simulink model "deep_pp"  (R2025b)
settings: Solver=FixedStepAuto  StartTime=0.0  StopTime=300  FixedStep=.01  RelTol=1e-3
undefined symbols (not defined in the file or in its folder): battery_builder_rtmsupport, gcbh
libraries: Batteries_lib x15, nesl_utility x5, fl_lib x4, ee_lib x1
(part 1 of 2)
settings Model: Creator=nhamb  LastModifiedBy=nhamb

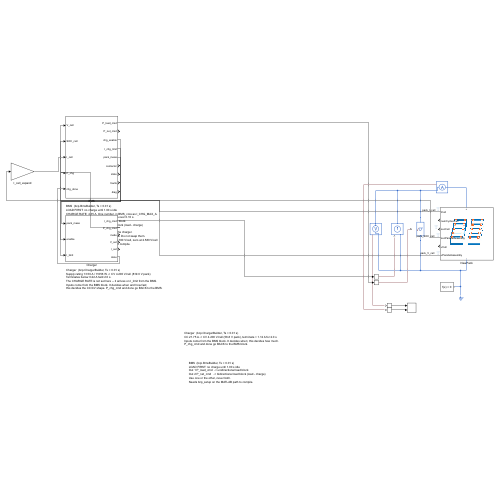
[thumbnail: Simulink's stored preview of the top-level diagram]
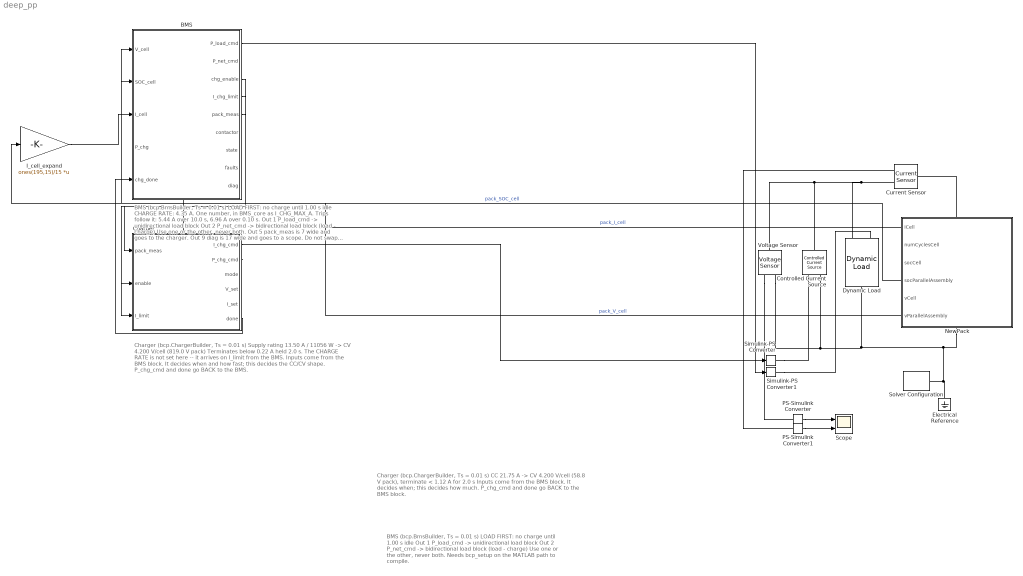
== system deep_pp ==
  note: BMS  (bcp.BmsBuilder, Ts = 0.01 s)
      | LOAD FIRST: no charge until 1.00 s idle
      | Out 1 P_load_cmd  -> unidirectional load block
      | Out 2 P_net_cmd   -> bidirectional load block (load - charge)
      | Use one or the other, never both.
      | Needs bcp_setup on the MATLAB path to compile.
  note: Charger  (bcp.ChargerBuilder, Ts = 0.01 s)
      | CC 21.75 A -> CV 4.200 V/cell (58.8 V pack), terminate < 1.12 A for 2.0 s
      | Inputs come from the BMS block. It decides when; this decides how much.
      | P_chg_cmd and done go BACK to the BMS block.
  note: BMS  (bcp.BmsBuilder, Ts = 0.01 s)
      | LOAD FIRST: no charge until 1.00 s idle
      | CHARGE RATE: 4.35 A. One number, in BMS_core as I_CHG_MAX_A.
      |   Trips follow it: 5.44 A over 10.0 s, 6.96 A over 0.10 s.
      | Out 1 P_load_cmd  -> unidirectional load block
      | Out 2 P_net_cmd   -> bidirectional load block (load - charge)
      | Use one or the other, never both.
      | Out 5 pack_meas is 7 wide and goes to the charger.
      | Out 9 diag is 17 wide and goes to a scope. Do not swap them.
      | DISCHARGE LIMITER: full load above 2.780 V/cell, zero at 2.580 V/cell
      | Needs bcp_setup on the MATLAB path to compile.
  note: Charger  (bcp.ChargerBuilder, Ts = 0.01 s)
      | Supply rating 13.50 A / 11056 W -> CV 4.200 V/cell (819.0 V pack)
      | Terminates below 0.22 A held 2.0 s.
      | The CHARGE RATE is not set here -- it arrives on I_limit from the BMS.
      | Inputs come from the BMS block. It decides when and how fast;
      | this decides the CC/CV shape. P_chg_cmd and done go BACK to the BMS.
  BMS : Subsystem
  Charger : Subsystem
  Controlled Current Source : fl_lib/Electrical/Electrical Sources/Controlled Current Source
  Current Sensor : fl_lib/Electrical/Electrical Sensors/Current Sensor
  Dynamic Load : ee_lib/Passive/Dynamic Load  load_type=ee.enum.dc_ac.dc  min_supply_voltage=20 V  pow_min=1e-3 W  G_reverse=1e-6 S  deltaV=1e-3 V  f0=60 Hz  Vrms_min=200 V  tau=0.01 s  Vrms_ini=300 V  Vang_ini=0 deg
      settings: InternalSimscapePortConfiguration="{\"Bottom\":[],\"Left\":[{\"id\":\"p\",\"label\":\"+\",\"type\":\"foundation.electrical.electrical\"}],\"Right\":[{\"id\":\"n\",\"label\":\"-\",\"type\":\"foundation.electrical.electrical\"}],\"Top\":[{\"id\":\"P\",\"label\":\"P\",\"type\":\"input\"}]}"
  Electrical Reference : fl_lib/Electrical/Electrical Elements/Electrical Reference
  I_cell_expand : Gain  Gain=ones(195,15)/15  Multiplication=Matrix(K*u)
  NewPack : Subsystem  LoadFcn=battery_builder_rtmsupport('loadfcn',gcbh);
      settings: CopyFcn=battery_builder_rtmsupport('copyfcn',gcbh);  PreCopyFcn=battery_builder_rtmsupport('precopyfcn',gcbh);  PreDeleteFcn=battery_builder_rtmsupport('predeletefcn',gcbh);  PortSchema="{\"entries\":[{\"content\":{\"sides\":[{\"content\":{\"connectorIds\":[\"LConn1\"]},\"type\":\"ConnectorPlacement.EquallySpacedRectSide\",\"uuid\":\"639f1e3e-b529-4ef3-8a0e-59dadedc297f\"},{\"content\":{\"connectorIds\":[\"RConn1\"],\"side\":\"RIGHT\"},\"type\":\"ConnectorPlacement.EquallySpacedRectSide\",\"uuid\":\"fd02ecdf-1885-4056-8ffe-a1dd80f7e2bb\"},{\"content\":{\"side\":\"TOP\"},\"type\":\"ConnectorPlacement.EquallySpacedRectSide\",\"uuid\":\"7ee78b50-8b8e-447f-8754-7e3c87fbecdf\"},{\"content\":{\"connectorIds\":[\"Out1\",\"Out2\",\"Out3\",\"Out4\",\"Out5\",\"Out6\"],\"side\":\"BOTTOM\"},\"type\":\"ConnectorPlacement.EquallySpacedRectSide\",\"uuid\":\"bf99fb64-3b35-4929-842b-dc936d21827d\"}]},\"type\":\"ConnectorPlacement.EquallySpacedConnector\",\"uuid\":\"bfe7ef6e-8305-4395-9b95-13fe458d8955\"}],\"packageUris\":[\"http://schema.mathworks.com/mf0/Connector/R2020b\"],\"version\":\"1.0\"}"
      mask Display: image('$imagefile')
  PS-Simulink Converter : nesl_utility/PS-Simulink Converter  PhysicalDomain=network_engine_domain  SubClassName=ps_output  LeftPortType=input  RightPortType=output  PseudoPeriodic=off  Frequencies=[]  VectorFormat=inherit  Unit=inherit  AffineConversion=off
  PS-Simulink Converter1 : nesl_utility/PS-Simulink Converter  PhysicalDomain=network_engine_domain  SubClassName=ps_output  LeftPortType=input  RightPortType=output  PseudoPeriodic=off  Frequencies=[]  VectorFormat=inherit  Unit=inherit  AffineConversion=off
  Scope : Scope  NumInputPorts=2
      settings: ActiveDisplayYMinimum=41.312958628712209  ActiveDisplayYMaximum=167.00529821946185
  Simulink-PS Converter : nesl_utility/Simulink-PS Converter  PhysicalDomain=network_engine_domain  SubClassName=ps_input  LeftPortType=input  RightPortType=output  PseudoPeriodic=off  Frequencies=[]  NoiseDistribution=none  NoiseParameters=[]  Unit=1  AffineConversion=off  FilteringAndDerivatives=provide  SimscapeFilterOrder=1  InputFilterTimeConstant=0.001  UdotUserProvided=0
  Simulink-PS Converter1 : nesl_utility/Simulink-PS Converter  PhysicalDomain=network_engine_domain  SubClassName=ps_input  LeftPortType=input  RightPortType=output  PseudoPeriodic=off  Frequencies=[]  NoiseDistribution=none  NoiseParameters=[]  Unit=1  AffineConversion=off  FilteringAndDerivatives=provide  SimscapeFilterOrder=1  InputFilterTimeConstant=0.001  UdotUserProvided=0
  Solver Configuration : nesl_utility/Solver Configuration  PhysicalDomain=network_engine_domain  SubClassName=solver  LeftPortType=input  RightPortType=generic  Tones=[]  Harmonics=[]  SimulateNoise=off  Profile=off  UseLocalSampling=off  EnableSwitchedLinearOptims=on  FrequencyDomain=off  UseCCode=off  RelTol=0.001  AbsTol=0.001  MinStep=1e-09  ToWorkspace=off  RevertToSquareIcSolve=off  NumHomotopyIterations=100  PhasorMode=off  PhasorModeNumHarmonics=1  ConsistencySolver=NEWTON_XTOL_AFTER_FTOL  IndexReductionMethod=DerivativeReplacement  DoDC=off  ResidualTolerance=1e-09  ConsistencyTolSource=GLOBAL  ConsistencyAbsTol=0.001  ConsistencyRelTol=0.001  ConsistencyTolFactor=0.001  UseLocalSolver=off  LocalSolverChoice=NE_BACKWARD_EULER_ADVANCER  ResolveIndetEquations=on  FunctionEvalNumThread=1  LocalSolverSampleTime=0.001  DoFixedCost=off  MaxNonlinIter=3  MaxModeIter=2  ComputeImpulses=off  ImpulseIterations=2  LinearAlgebra=auto  LinearAlgebraNumThread=0  EquationFormulation=NE_TIME_EF  DelaysMemoryBudget=1024  AutomaticFiltering=on  FilteringTimeConstant=0.001  PartitionStorageMethod=AS_NEEDED  PartitionMemoryBudget=1024  PartitionMethod=ROBUST  MultibodyUseLocalSolver=off  MultibodyLocalSolverChoice=ODE1  MultibodyLocalSolverSampleTime=0.001
  Voltage Sensor : fl_lib/Electrical/Electrical Sensors/Voltage Sensor
  wires:
  PS-Simulink Converter1/1 -> Scope/2
  PS-Simulink Converter/1 -> Scope/1
  BMS/5(pack_meas) -> Charger/1(pack_meas)
  BMS/3(chg_enable) -> Charger/2(enable)
  BMS/4(I_chg_limit) -> Charger/3(I_limit)
  Charger/2(P_chg_cmd) -> BMS/4(P_chg)
  Charger/6(done) -> BMS/5(chg_done)
  NewPack/1(iCell) -> I_cell_expand/1  "pack_I_cell"
  I_cell_expand/1 -> BMS/3(I_cell)
  NewPack/6(vParallelAssembly) -> BMS/1(V_cell)  "pack_V_cell"
  NewPack/4(socParallelAssembly) -> BMS/2(SOC_cell)  "pack_SOC_cell"
  BMS/1(P_load_cmd) -> Simulink-PS Converter1/1
  Charger/1(I_chg_cmd) -> Simulink-PS Converter/1
  connections:
  Controlled Current Source/RConn2 -- Solver Configuration/RConn1 -- Electrical Reference/LConn1 -- NewPack/RConn1 -- Dynamic Load/RConn1 -- Voltage Sensor/RConn2
  Current Sensor/RConn2 -- Dynamic Load/LConn1 -- Voltage Sensor/LConn1 -- Controlled Current Source/LConn1
  NewPack/LConn1 -- Current Sensor/LConn1
  Simulink-PS Converter/RConn1 -- Controlled Current Source/RConn1
  Simulink-PS Converter1/RConn1 -- Dynamic Load/LConn2
  Voltage Sensor/RConn1 -- PS-Simulink Converter/LConn1
  Current Sensor/RConn1 -- PS-Simulink Converter1/LConn1

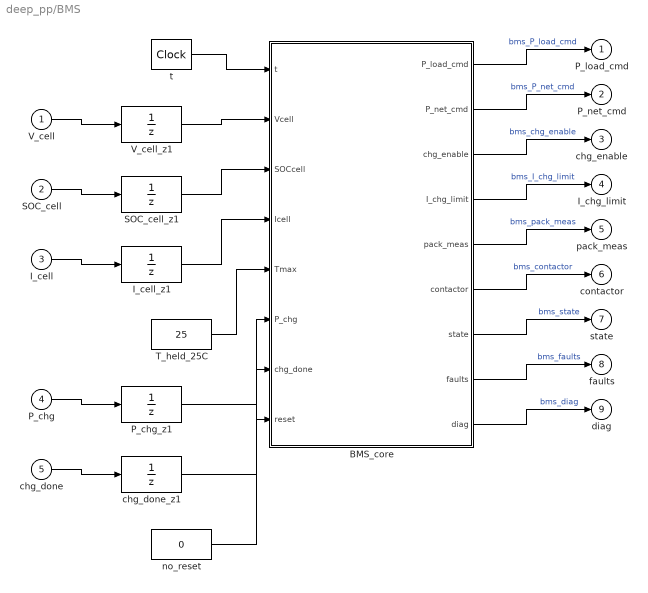
== system deep_pp/BMS ==
  V_cell : Inport
  SOC_cell : Inport  Port=2
  I_cell : Inport  Port=3
  P_chg : Inport  Port=4
  chg_done : Inport  Port=5
  BMS_core : MATLAB Function  TreatAsAtomicUnit=on
  I_cell_z1 : UnitDelay  SampleTime=0.01  HasFrameUpgradeWarning=on
  P_chg_z1 : UnitDelay  SampleTime=0.01  HasFrameUpgradeWarning=on
  SOC_cell_z1 : UnitDelay  InitialCondition=0.5  SampleTime=0.01  HasFrameUpgradeWarning=on
  T_held_25C : Constant  Value=25
  V_cell_z1 : UnitDelay  InitialCondition=3.575  SampleTime=0.01  HasFrameUpgradeWarning=on
  chg_done_z1 : UnitDelay  SampleTime=0.01  HasFrameUpgradeWarning=on
  no_reset : Constant  Value=0
  t : DigitalClock  SampleTime=0.01
  P_load_cmd : Outport
  P_net_cmd : Outport  Port=2
  chg_enable : Outport  Port=3
  I_chg_limit : Outport  Port=4
  pack_meas : Outport  Port=5
  contactor : Outport  Port=6
  state : Outport  Port=7
  faults : Outport  Port=8
  diag : Outport  Port=9
  wires:
  t/1 -> BMS_core/1(t)
  V_cell/1 -> V_cell_z1/1
  V_cell_z1/1 -> BMS_core/2(Vcell)
  SOC_cell/1 -> SOC_cell_z1/1
  SOC_cell_z1/1 -> BMS_core/3(SOCcell)
  I_cell/1 -> I_cell_z1/1
  I_cell_z1/1 -> BMS_core/4(Icell)
  T_held_25C/1 -> BMS_core/5(Tmax)
  P_chg/1 -> P_chg_z1/1
  P_chg_z1/1 -> BMS_core/6(P_chg)
  chg_done/1 -> chg_done_z1/1
  chg_done_z1/1 -> BMS_core/7(chg_done)
  no_reset/1 -> BMS_core/8(reset)
  BMS_core/1(P_load_cmd) -> P_load_cmd/1  "bms_P_load_cmd"
  BMS_core/2(P_net_cmd) -> P_net_cmd/1  "bms_P_net_cmd"
  BMS_core/3(chg_enable) -> chg_enable/1  "bms_chg_enable"
  BMS_core/4(I_chg_limit) -> I_chg_limit/1  "bms_I_chg_limit"
  BMS_core/5(pack_meas) -> pack_meas/1  "bms_pack_meas"
  BMS_core/6(contactor) -> contactor/1  "bms_contactor"
  BMS_core/7(state) -> state/1  "bms_state"
  BMS_core/8(faults) -> faults/1  "bms_faults"
  BMS_core/9(diag) -> diag/1  "bms_diag"

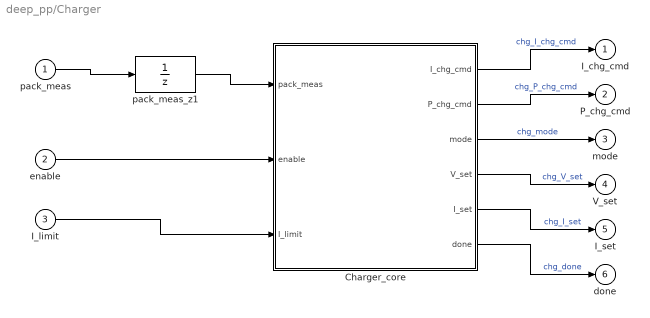
== system deep_pp/Charger ==
  pack_meas : Inport
  enable : Inport  Port=2
  I_limit : Inport  Port=3
  Charger_core : MATLAB Function  TreatAsAtomicUnit=on
  pack_meas_z1 : UnitDelay  InitialCondition=[819;4.2;4.2;1;1;1;0]  SampleTime=0.01  HasFrameUpgradeWarning=on
  I_chg_cmd : Outport
  P_chg_cmd : Outport  Port=2
  mode : Outport  Port=3
  V_set : Outport  Port=4
  I_set : Outport  Port=5
  done : Outport  Port=6
  wires:
  pack_meas/1 -> pack_meas_z1/1
  pack_meas_z1/1 -> Charger_core/1(pack_meas)
  enable/1 -> Charger_core/2(enable)
  I_limit/1 -> Charger_core/3(I_limit)
  Charger_core/1(I_chg_cmd) -> I_chg_cmd/1  "chg_I_chg_cmd"
  Charger_core/2(P_chg_cmd) -> P_chg_cmd/1  "chg_P_chg_cmd"
  Charger_core/3(mode) -> mode/1  "chg_mode"
  Charger_core/4(V_set) -> V_set/1  "chg_V_set"
  Charger_core/5(I_set) -> I_set/1  "chg_I_set"
  Charger_core/6(done) -> done/1  "chg_done"

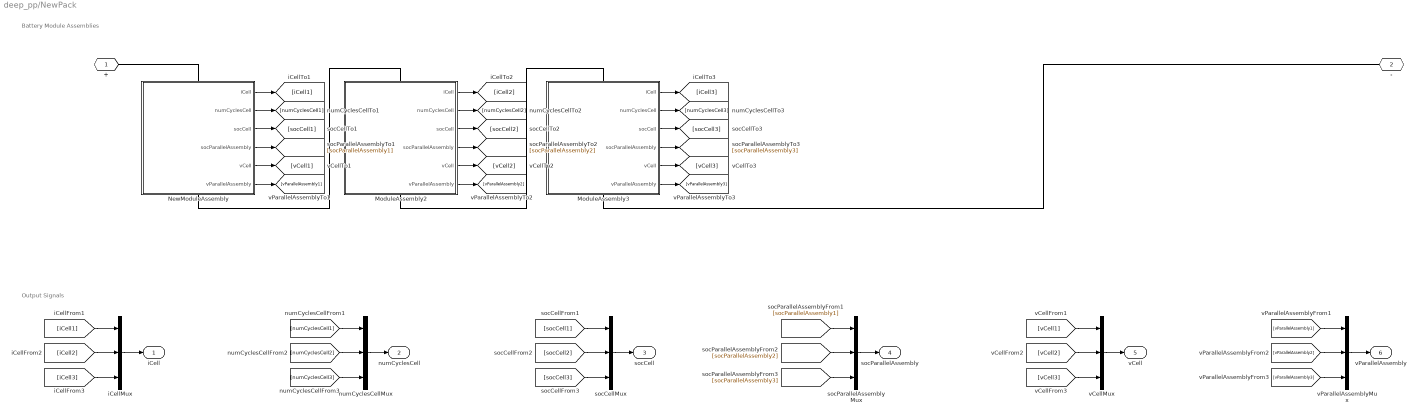
== system deep_pp/NewPack ==
  note: Output Signals
  note: Battery Module Assemblies
  ModuleAssembly2 : Subsystem  LoadFcn=battery_builder_rtmsupport('loadfcn',gcbh);
      settings: CopyFcn=battery_builder_rtmsupport('copyfcn',gcbh);  PreCopyFcn=battery_builder_rtmsupport('precopyfcn',gcbh);  PreDeleteFcn=battery_builder_rtmsupport('predeletefcn',gcbh);  PortSchema="{\"entries\":[{\"content\":{\"sides\":[{\"content\":{\"connectorIds\":[\"LConn1\"]},\"type\":\"ConnectorPlacement.EquallySpacedRectSide\",\"uuid\":\"639f1e3e-b529-4ef3-8a0e-59dadedc297f\"},{\"content\":{\"connectorIds\":[\"RConn1\"],\"side\":\"RIGHT\"},\"type\":\"ConnectorPlacement.EquallySpacedRectSide\",\"uuid\":\"fd02ecdf-1885-4056-8ffe-a1dd80f7e2bb\"},{\"content\":{\"side\":\"TOP\"},\"type\":\"ConnectorPlacement.EquallySpacedRectSide\",\"uuid\":\"7ee78b50-8b8e-447f-8754-7e3c87fbecdf\"},{\"content\":{\"connectorIds\":[\"Out1\",\"Out2\",\"Out3\",\"Out4\",\"Out5\",\"Out6\"],\"side\":\"BOTTOM\"},\"type\":\"ConnectorPlacement.EquallySpacedRectSide\",\"uuid\":\"6ddc3ac7-a805-4d8e-a52b-67f31048dafb\"}]},\"type\":\"ConnectorPlacement.EquallySpacedConnector\",\"uuid\":\"bfe7ef6e-8305-4395-9b95-13fe458d8955\"}],\"packageUris\":[\"http://schema.mathworks.com/mf0/Connector/R2020b\"],\"version\":\"1.0\"}"
      mask Display: image('$imagefile')
  ModuleAssembly3 : Subsystem  LoadFcn=battery_builder_rtmsupport('loadfcn',gcbh);
      settings: CopyFcn=battery_builder_rtmsupport('copyfcn',gcbh);  PreCopyFcn=battery_builder_rtmsupport('precopyfcn',gcbh);  PreDeleteFcn=battery_builder_rtmsupport('predeletefcn',gcbh);  PortSchema="{\"entries\":[{\"content\":{\"sides\":[{\"content\":{\"connectorIds\":[\"LConn1\"]},\"type\":\"ConnectorPlacement.EquallySpacedRectSide\",\"uuid\":\"639f1e3e-b529-4ef3-8a0e-59dadedc297f\"},{\"content\":{\"connectorIds\":[\"RConn1\"],\"side\":\"RIGHT\"},\"type\":\"ConnectorPlacement.EquallySpacedRectSide\",\"uuid\":\"fd02ecdf-1885-4056-8ffe-a1dd80f7e2bb\"},{\"content\":{\"side\":\"TOP\"},\"type\":\"ConnectorPlacement.EquallySpacedRectSide\",\"uuid\":\"7ee78b50-8b8e-447f-8754-7e3c87fbecdf\"},{\"content\":{\"connectorIds\":[\"Out1\",\"Out2\",\"Out3\",\"Out4\",\"Out5\",\"Out6\"],\"side\":\"BOTTOM\"},\"type\":\"ConnectorPlacement.EquallySpacedRectSide\",\"uuid\":\"6ddc3ac7-a805-4d8e-a52b-67f31048dafb\"}]},\"type\":\"ConnectorPlacement.EquallySpacedConnector\",\"uuid\":\"bfe7ef6e-8305-4395-9b95-13fe458d8955\"}],\"packageUris\":[\"http://schema.mathworks.com/mf0/Connector/R2020b\"],\"version\":\"1.0\"}"
      mask Display: image('moduleAssembly_1.JPG');
  NewModuleAssembly : Subsystem  LoadFcn=battery_builder_rtmsupport('loadfcn',gcbh);
      settings: CopyFcn=battery_builder_rtmsupport('copyfcn',gcbh);  PreCopyFcn=battery_builder_rtmsupport('precopyfcn',gcbh);  PreDeleteFcn=battery_builder_rtmsupport('predeletefcn',gcbh);  PortSchema="{\"entries\":[{\"content\":{\"sides\":[{\"content\":{\"connectorIds\":[\"LConn1\"]},\"type\":\"ConnectorPlacement.EquallySpacedRectSide\",\"uuid\":\"639f1e3e-b529-4ef3-8a0e-59dadedc297f\"},{\"content\":{\"connectorIds\":[\"RConn1\"],\"side\":\"RIGHT\"},\"type\":\"ConnectorPlacement.EquallySpacedRectSide\",\"uuid\":\"fd02ecdf-1885-4056-8ffe-a1dd80f7e2bb\"},{\"content\":{\"side\":\"TOP\"},\"type\":\"ConnectorPlacement.EquallySpacedRectSide\",\"uuid\":\"7ee78b50-8b8e-447f-8754-7e3c87fbecdf\"},{\"content\":{\"connectorIds\":[\"Out1\",\"Out2\",\"Out3\",\"Out4\",\"Out5\",\"Out6\"],\"side\":\"BOTTOM\"},\"type\":\"ConnectorPlacement.EquallySpacedRectSide\",\"uuid\":\"6ddc3ac7-a805-4d8e-a52b-67f31048dafb\"}]},\"type\":\"ConnectorPlacement.EquallySpacedConnector\",\"uuid\":\"bfe7ef6e-8305-4395-9b95-13fe458d8955\"}],\"packageUris\":[\"http://schema.mathworks.com/mf0/Connector/R2020b\"],\"version\":\"1.0\"}"
      mask Display: image('moduleAssembly_2.JPG');
  iCellMux : Mux  Inputs=3
  numCyclesCellMux : Mux  Inputs=3
  socCellMux : Mux  Inputs=3
  socParallelAssemblyMux : Mux  Inputs=3
  vCellMux : Mux  Inputs=3
  vParallelAssemblyMux : Mux  Inputs=3
  + : PMIOPort  Side=Left
  - : PMIOPort  Port=2  Side=Right
  iCell : Outport
  numCyclesCell : Outport  Port=2
  socCell : Outport  Port=3
  socParallelAssembly : Outport  Port=4
  vCell : Outport  Port=5
  vParallelAssembly : Outport  Port=6
  wires:
  [vParallelAssembly3] -> vParallelAssemblyMux/3
  ModuleAssembly3/6(vParallelAssembly) -> [vParallelAssembly3]
  [vCell3] -> vCellMux/3
  ModuleAssembly3/5(vCell) -> [vCell3]
  [socParallelAssembly3] -> socParallelAssemblyMux/3
  ModuleAssembly3/4(socParallelAssembly) -> [socParallelAssembly3]
  [socCell3] -> socCellMux/3
  ModuleAssembly3/3(socCell) -> [socCell3]
  [numCyclesCell3] -> numCyclesCellMux/3
  ModuleAssembly3/2(numCyclesCell) -> [numCyclesCell3]
  [iCell3] -> iCellMux/3
  ModuleAssembly3/1(iCell) -> [iCell3]
  [vParallelAssembly2] -> vParallelAssemblyMux/2
  ModuleAssembly2/6(vParallelAssembly) -> [vParallelAssembly2]
  [vCell2] -> vCellMux/2
  ModuleAssembly2/5(vCell) -> [vCell2]
  [socParallelAssembly2] -> socParallelAssemblyMux/2
  ModuleAssembly2/4(socParallelAssembly) -> [socParallelAssembly2]
  [socCell2] -> socCellMux/2
  ModuleAssembly2/3(socCell) -> [socCell2]
  [numCyclesCell2] -> numCyclesCellMux/2
  ModuleAssembly2/2(numCyclesCell) -> [numCyclesCell2]
  [iCell2] -> iCellMux/2
  ModuleAssembly2/1(iCell) -> [iCell2]
  [vParallelAssembly1] -> vParallelAssemblyMux/1
  vParallelAssemblyMux/1 -> vParallelAssembly/1
  NewModuleAssembly/6(vParallelAssembly) -> [vParallelAssembly1]
  [vCell1] -> vCellMux/1
  vCellMux/1 -> vCell/1
  NewModuleAssembly/5(vCell) -> [vCell1]
  [socParallelAssembly1] -> socParallelAssemblyMux/1
  socParallelAssemblyMux/1 -> socParallelAssembly/1
  NewModuleAssembly/4(socParallelAssembly) -> [socParallelAssembly1]
  [socCell1] -> socCellMux/1
  socCellMux/1 -> socCell/1
  NewModuleAssembly/3(socCell) -> [socCell1]
  [numCyclesCell1] -> numCyclesCellMux/1
  numCyclesCellMux/1 -> numCyclesCell/1
  NewModuleAssembly/2(numCyclesCell) -> [numCyclesCell1]
  [iCell1] -> iCellMux/1
  iCellMux/1 -> iCell/1
  NewModuleAssembly/1(iCell) -> [iCell1]
  connections:
  ModuleAssembly3/RConn1 -- -/RConn1
  NewModuleAssembly/LConn1 -- +/RConn1
  ModuleAssembly3/LConn1 -- ModuleAssembly2/RConn1
  ModuleAssembly2/LConn1 -- NewModuleAssembly/RConn1

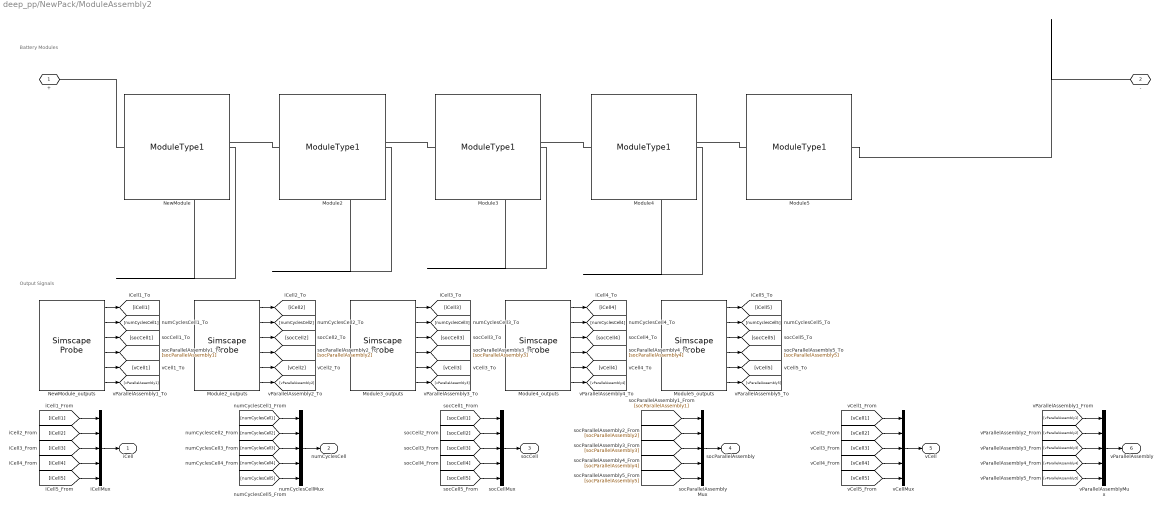
== system deep_pp/NewPack/ModuleAssembly2 ==
  note: Battery Modules
  note: Output Signals
  Module{2..5} (4 alike) : Batteries_lib/Modules/ModuleType1  SOC_vecCell=[0, .01, .02, .03, .04, .05, .06, .07, .08, .09, .1, .11, .12, .13, .14, .15, .16, .17, .18, .19, .2, .21, .22, .23, .24, .25, .26, .27, .28, .29, .3, .31, .32, .33, .34, .35, .36, .37, .38, .39, .4, .41, .42, .43, .44, .45, .46, .47, .48, .49, .5, .51, .52, .53, .54, .55, .56, .57, .58, .59, .6, .61, .62, .63, .64, .65, .66, .67, .68, .69, .7, .71, .72, .73, .74, .75, .76, .77, .78, .79, .8, .81, .82, .83, .84, .85, .86, .87, .88, .89, .9, .91, .92, .93, .94, .95, .96, .97, .98, .99, 1]  V0_vecCell=[3.17242, 3.18272, 3.19302, 3.20331, 3.21361, 3.22391, 3.23421, 3.24451, 3.25481, 3.2651, 3.2754, 3.2857, 3.296, 3.3063, 3.31659, 3.32689, 3.33719, 3.34749, 3.35779, 3.36809, 3.37838, 3.38868, 3.39898, 3.40928, 3.41958, 3.42988, 3.44017, 3.45047, 3.46077, 3.47107, 3.48137, 3.49166, 3.50196, 3.51226, 3.52256, 3.53286, 3.54316, 3.55345, 3.56375, 3.57405, 3.58435, 3.59465, 3.60495, 3.61524, 3.62554, 3.63584, 3.64614, 3.65644, 3.66673, 3.67703, 3.68733, 3.69763, 3.71041, 3.72113, 3.72997, 3.73882, 3.74912, 3.75936, 3.76951, 3.7791, 3.78865, 3.79787, 3.80709, 3.8161, 3.82509, 3.83409, 3.84308, 3.85207, 3.86107, 3.87006, 3.87901, 3.88831, 3.89824, 3.90887, 3.91951, 3.93012, 3.94073, 3.95138, 3.96184, 3.97226, 3.98268, 3.99311, 4.0032, 4.01221, 4.01944, 4.02668, 4.03286, 4.03874, 4.04383, 4.0488, 4.05377, 4.05873, 4.06312, 4.06753, 4.07333, 4.08117, 4.08904, 4.09911, 4.11111, 4.13802, 4.16831] V  V_rangeCell=[2.25, Inf] V  R0_vecCell=[.02095, .01921, .01774, .0166, .01557, .01469, .01398, .01338, .01283, .01239, .01196, .01155, .01116, .01079, .01042, .01007, .00974, .00949, .00924, .009, .00876, .00855, .00843, .00832, .00826, .00825, .00825, .00826, .00827, .00828, .0083, .00834, .00838, .00842, .00848, .00855, .00863, .00871, .00879, .00887, .00895, .00903, .00911, .00918, .00925, .00931, .00938, .00946, .00953, .00961, .00968, .00976, .00991, .01, .01003, .01006, .01013, .01022, .0103, .01037, .01043, .01049, .01055, .01061, .01066, .01072, .01077, .01082, .01088, .01093, .01099, .01105, .01114, .01125, .01136, .01148, .01161, .01175, .01188, .01202, .01215, .01228, .01241, .01253, .01261, .01269, .01275, .0128, .01285, .01289, .01294, .01298, .01296, .01292, .01292, .01288, .01282, .0128, .01232, .01214, .00952] Ohm  AHCell=4.493 A*hr  extrapolation_optionCell=simscape.enum.extrapolation.nearest  P=1  S=13  iCell_specify=off  iCell_priority=None  iCell=0 A  iCell_nominal_specify=off  iCell_nominal_value=1  iCell_nominal_unit=A  vCell_specify=off  vCell_priority=None  vCell=0 V  vCell_nominal_specify=off  vCell_nominal_value=1  vCell_nominal_unit=V  socCell_specify=on  socCell_priority=High  socCell=0.08  socCell_nominal_specify=off  socCell_nominal_value=1  socCell_nominal_unit=1  numCyclesCell_specify=off  numCyclesCell_priority=High  numCyclesCell=0  numCyclesCell_nominal_specify=off  numCyclesCell_nominal_value=1  numCyclesCell_nominal_unit=1  vParallelAssembly_specify=off  vParallelAssembly_priority=None  vParallelAssembly=repmat(0, 13, 1) V  vParallelAssembly_nominal_specify=off  vParallelAssembly_nominal_value=1  vParallelAssembly_nominal_unit=V  socParallelAssembly_specify=off  socParallelAssembly_priority=None  socParallelAssembly=repmat(1, 13, 1)  socParallelAssembly_nominal_specify=off  socParallelAssembly_nominal_value=1  socParallelAssembly_nominal_unit=1
      settings: InternalSimscapePortConfiguration="{\"Bottom\":[{\"id\":\"n\",\"label\":\"-\",\"type\":\"foundation.electrical.electrical\"}],\"Left\":[],\"Right\":[],\"Top\":[{\"id\":\"p\",\"label\":\"+\",\"type\":\"foundation.electrical.electrical\"}]}"
  Module2_outputs : SimscapeProbe  BoundBlock=53  Variables="{\"iCell\":{\"Probing\":\"ON\"},\"numCyclesCell\":{\"Probing\":\"ON\"},\"socCell\":{\"Probing\":\"ON\"},\"socParallelAssembly\":{\"Probing\":\"ON\"},\"vCell\":{\"Probing\":\"ON\"},\"vParallelAssembly\":{\"Probing\":\"ON\"}}"
  Module3_outputs : SimscapeProbe  BoundBlock=55  Variables="{\"iCell\":{\"Probing\":\"ON\"},\"numCyclesCell\":{\"Probing\":\"ON\"},\"socCell\":{\"Probing\":\"ON\"},\"socParallelAssembly\":{\"Probing\":\"ON\"},\"vCell\":{\"Probing\":\"ON\"},\"vParallelAssembly\":{\"Probing\":\"ON\"}}"
  Module4_outputs : SimscapeProbe  BoundBlock=57  Variables="{\"iCell\":{\"Probing\":\"ON\"},\"numCyclesCell\":{\"Probing\":\"ON\"},\"socCell\":{\"Probing\":\"ON\"},\"socParallelAssembly\":{\"Probing\":\"ON\"},\"vCell\":{\"Probing\":\"ON\"},\"vParallelAssembly\":{\"Probing\":\"ON\"}}"
  Module5_outputs : SimscapeProbe  BoundBlock=59  Variables="{\"iCell\":{\"Probing\":\"ON\"},\"numCyclesCell\":{\"Probing\":\"ON\"},\"socCell\":{\"Probing\":\"ON\"},\"socParallelAssembly\":{\"Probing\":\"ON\"},\"vCell\":{\"Probing\":\"ON\"},\"vParallelAssembly\":{\"Probing\":\"ON\"}}"
  NewModule : Batteries_lib/Modules/ModuleType1  SOC_vecCell=[0, .01, .02, .03, .04, .05, .06, .07, .08, .09, .1, .11, .12, .13, .14, .15, .16, .17, .18, .19, .2, .21, .22, .23, .24, .25, .26, .27, .28, .29, .3, .31, .32, .33, .34, .35, .36, .37, .38, .39, .4, .41, .42, .43, .44, .45, .46, .47, .48, .49, .5, .51, .52, .53, .54, .55, .56, .57, .58, .59, .6, .61, .62, .63, .64, .65, .66, .67, .68, .69, .7, .71, .72, .73, .74, .75, .76, .77, .78, .79, .8, .81, .82, .83, .84, .85, .86, .87, .88, .89, .9, .91, .92, .93, .94, .95, .96, .97, .98, .99, 1]  V0_vecCell=[3.17242, 3.18272, 3.19302, 3.20331, 3.21361, 3.22391, 3.23421, 3.24451, 3.25481, 3.2651, 3.2754, 3.2857, 3.296, 3.3063, 3.31659, 3.32689, 3.33719, 3.34749, 3.35779, 3.36809, 3.37838, 3.38868, 3.39898, 3.40928, 3.41958, 3.42988, 3.44017, 3.45047, 3.46077, 3.47107, 3.48137, 3.49166, 3.50196, 3.51226, 3.52256, 3.53286, 3.54316, 3.55345, 3.56375, 3.57405, 3.58435, 3.59465, 3.60495, 3.61524, 3.62554, 3.63584, 3.64614, 3.65644, 3.66673, 3.67703, 3.68733, 3.69763, 3.71041, 3.72113, 3.72997, 3.73882, 3.74912, 3.75936, 3.76951, 3.7791, 3.78865, 3.79787, 3.80709, 3.8161, 3.82509, 3.83409, 3.84308, 3.85207, 3.86107, 3.87006, 3.87901, 3.88831, 3.89824, 3.90887, 3.91951, 3.93012, 3.94073, 3.95138, 3.96184, 3.97226, 3.98268, 3.99311, 4.0032, 4.01221, 4.01944, 4.02668, 4.03286, 4.03874, 4.04383, 4.0488, 4.05377, 4.05873, 4.06312, 4.06753, 4.07333, 4.08117, 4.08904, 4.09911, 4.11111, 4.13802, 4.16831] V  V_rangeCell=[2.25, Inf] V  R0_vecCell=[.02095, .01921, .01774, .0166, .01557, .01469, .01398, .01338, .01283, .01239, .01196, .01155, .01116, .01079, .01042, .01007, .00974, .00949, .00924, .009, .00876, .00855, .00843, .00832, .00826, .00825, .00825, .00826, .00827, .00828, .0083, .00834, .00838, .00842, .00848, .00855, .00863, .00871, .00879, .00887, .00895, .00903, .00911, .00918, .00925, .00931, .00938, .00946, .00953, .00961, .00968, .00976, .00991, .01, .01003, .01006, .01013, .01022, .0103, .01037, .01043, .01049, .01055, .01061, .01066, .01072, .01077, .01082, .01088, .01093, .01099, .01105, .01114, .01125, .01136, .01148, .01161, .01175, .01188, .01202, .01215, .01228, .01241, .01253, .01261, .01269, .01275, .0128, .01285, .01289, .01294, .01298, .01296, .01292, .01292, .01288, .01282, .0128, .01232, .01214, .00952] Ohm  AHCell=4.493 A*hr  extrapolation_optionCell=simscape.enum.extrapolation.nearest  P=1  S=13  iCell_specify=off  iCell_priority=None  iCell=0 A  iCell_nominal_specify=off  iCell_nominal_value=1  iCell_nominal_unit=A  vCell_specify=off  vCell_priority=None  vCell=0 V  vCell_nominal_specify=off  vCell_nominal_value=1  vCell_nominal_unit=V  socCell_specify=on  socCell_priority=High  socCell=0.08  socCell_nominal_specify=off  socCell_nominal_value=1  socCell_nominal_unit=1  numCyclesCell_specify=off  numCyclesCell_priority=High  numCyclesCell=0  numCyclesCell_nominal_specify=off  numCyclesCell_nominal_value=1  numCyclesCell_nominal_unit=1  vParallelAssembly_specify=off  vParallelAssembly_priority=None  vParallelAssembly=repmat(0, 13, 1) V  vParallelAssembly_nominal_specify=off  vParallelAssembly_nominal_value=1  vParallelAssembly_nominal_unit=V  socParallelAssembly_specify=off  socParallelAssembly_priority=None  socParallelAssembly=repmat(1, 13, 1)  socParallelAssembly_nominal_specify=off  socParallelAssembly_nominal_value=1  socParallelAssembly_nominal_unit=1
      settings: InternalSimscapePortConfiguration="{\"Bottom\":[{\"id\":\"n\",\"label\":\"-\",\"type\":\"foundation.electrical.electrical\"}],\"Left\":[],\"Right\":[],\"Top\":[{\"id\":\"p\",\"label\":\"+\",\"type\":\"foundation.electrical.electrical\"}]}"
  NewModule_outputs : SimscapeProbe  BoundBlock=61  Variables="{\"iCell\":{\"Probing\":\"ON\"},\"numCyclesCell\":{\"Probing\":\"ON\"},\"socCell\":{\"Probing\":\"ON\"},\"socParallelAssembly\":{\"Probing\":\"ON\"},\"vCell\":{\"Probing\":\"ON\"},\"vParallelAssembly\":{\"Probing\":\"ON\"}}"
  iCellMux : Mux  Inputs=5
  numCyclesCellMux : Mux  Inputs=5
  socCellMux : Mux  Inputs=5
  socParallelAssemblyMux : Mux  Inputs=5
  vCellMux : Mux  Inputs=5
  vParallelAssemblyMux : Mux  Inputs=5
  + : PMIOPort  Side=Left
  - : PMIOPort  Port=2  Side=Right
  iCell : Outport
  numCyclesCell : Outport  Port=2
  socCell : Outport  Port=3
  socParallelAssembly : Outport  Port=4
  vCell : Outport  Port=5
  vParallelAssembly : Outport  Port=6
  wires:
  NewModule_outputs/1 -> [iCell1]
  iCellMux/1 -> iCell/1
  [iCell1] -> iCellMux/1
  NewModule_outputs/2 -> [numCyclesCell1]
  numCyclesCellMux/1 -> numCyclesCell/1
  [numCyclesCell1] -> numCyclesCellMux/1
  NewModule_outputs/3 -> [socCell1]
  socCellMux/1 -> socCell/1
  [socCell1] -> socCellMux/1
  NewModule_outputs/4 -> [socParallelAssembly1]
  socParallelAssemblyMux/1 -> socParallelAssembly/1
  [socParallelAssembly1] -> socParallelAssemblyMux/1
  NewModule_outputs/5 -> [vCell1]
  vCellMux/1 -> vCell/1
  [vCell1] -> vCellMux/1
  NewModule_outputs/6 -> [vParallelAssembly1]
  vParallelAssemblyMux/1 -> vParallelAssembly/1
  [vParallelAssembly1] -> vParallelAssemblyMux/1
  Module2_outputs/1 -> [iCell2]
  [iCell2] -> iCellMux/2
  Module2_outputs/2 -> [numCyclesCell2]
  [numCyclesCell2] -> numCyclesCellMux/2
  Module2_outputs/3 -> [socCell2]
  [socCell2] -> socCellMux/2
  Module2_outputs/4 -> [socParallelAssembly2]
  [socParallelAssembly2] -> socParallelAssemblyMux/2
  Module2_outputs/5 -> [vCell2]
  [vCell2] -> vCellMux/2
  Module2_outputs/6 -> [vParallelAssembly2]
  [vParallelAssembly2] -> vParallelAssemblyMux/2
  Module3_outputs/1 -> [iCell3]
  [iCell3] -> iCellMux/3
  Module3_outputs/2 -> [numCyclesCell3]
  [numCyclesCell3] -> numCyclesCellMux/3
  Module3_outputs/3 -> [socCell3]
  [socCell3] -> socCellMux/3
  Module3_outputs/4 -> [socParallelAssembly3]
  [socParallelAssembly3] -> socParallelAssemblyMux/3
  Module3_outputs/5 -> [vCell3]
  [vCell3] -> vCellMux/3
  Module3_outputs/6 -> [vParallelAssembly3]
  [vParallelAssembly3] -> vParallelAssemblyMux/3
  Module4_outputs/1 -> [iCell4]
  [iCell4] -> iCellMux/4
  Module4_outputs/2 -> [numCyclesCell4]
  [numCyclesCell4] -> numCyclesCellMux/4
  Module4_outputs/3 -> [socCell4]
  [socCell4] -> socCellMux/4
  Module4_outputs/4 -> [socParallelAssembly4]
  [socParallelAssembly4] -> socParallelAssemblyMux/4
  Module4_outputs/5 -> [vCell4]
  [vCell4] -> vCellMux/4
  Module4_outputs/6 -> [vParallelAssembly4]
  [vParallelAssembly4] -> vParallelAssemblyMux/4
  Module5_outputs/1 -> [iCell5]
  [iCell5] -> iCellMux/5
  Module5_outputs/2 -> [numCyclesCell5]
  [numCyclesCell5] -> numCyclesCellMux/5
  Module5_outputs/3 -> [socCell5]
  [socCell5] -> socCellMux/5
  Module5_outputs/4 -> [socParallelAssembly5]
  [socParallelAssembly5] -> socParallelAssemblyMux/5
  Module5_outputs/5 -> [vCell5]
  [vCell5] -> vCellMux/5
  Module5_outputs/6 -> [vParallelAssembly5]
  [vParallelAssembly5] -> vParallelAssemblyMux/5
  connections:
  Module2/LConn1 -- NewModule/RConn1
  Module3/LConn1 -- Module2/RConn1
  Module4/LConn1 -- Module3/RConn1
  Module5/LConn1 -- Module4/RConn1
  NewModule/LConn1 -- +/RConn1
  Module5/RConn1 -- -/RConn1

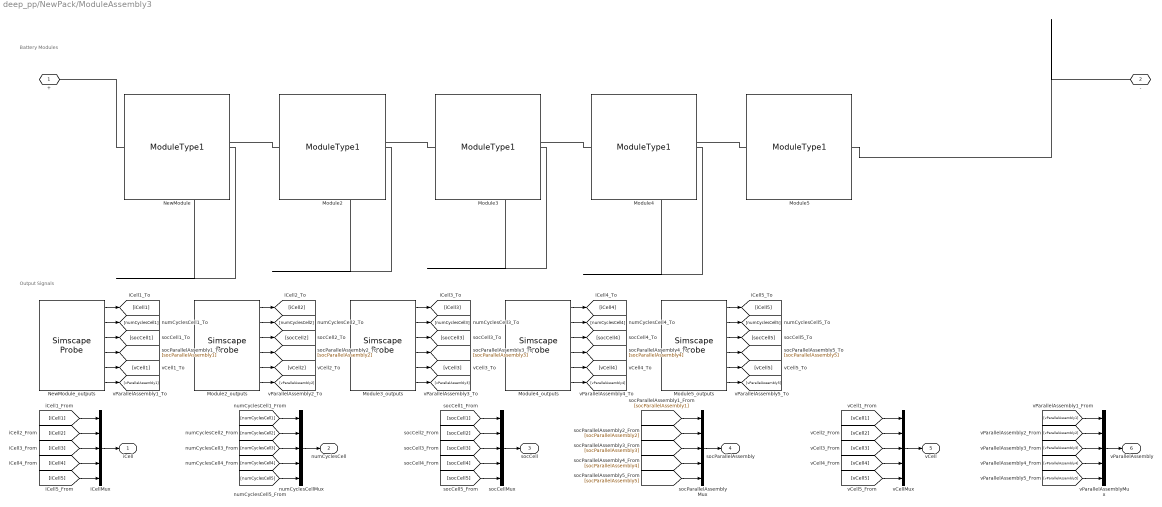
== system deep_pp/NewPack/ModuleAssembly3 ==
  note: Battery Modules
  note: Output Signals
  Module{2..5} (4 alike) : Batteries_lib/Modules/ModuleType1  SOC_vecCell=[0, .01, .02, .03, .04, .05, .06, .07, .08, .09, .1, .11, .12, .13, .14, .15, .16, .17, .18, .19, .2, .21, .22, .23, .24, .25, .26, .27, .28, .29, .3, .31, .32, .33, .34, .35, .36, .37, .38, .39, .4, .41, .42, .43, .44, .45, .46, .47, .48, .49, .5, .51, .52, .53, .54, .55, .56, .57, .58, .59, .6, .61, .62, .63, .64, .65, .66, .67, .68, .69, .7, .71, .72, .73, .74, .75, .76, .77, .78, .79, .8, .81, .82, .83, .84, .85, .86, .87, .88, .89, .9, .91, .92, .93, .94, .95, .96, .97, .98, .99, 1]  V0_vecCell=[3.17242, 3.18272, 3.19302, 3.20331, 3.21361, 3.22391, 3.23421, 3.24451, 3.25481, 3.2651, 3.2754, 3.2857, 3.296, 3.3063, 3.31659, 3.32689, 3.33719, 3.34749, 3.35779, 3.36809, 3.37838, 3.38868, 3.39898, 3.40928, 3.41958, 3.42988, 3.44017, 3.45047, 3.46077, 3.47107, 3.48137, 3.49166, 3.50196, 3.51226, 3.52256, 3.53286, 3.54316, 3.55345, 3.56375, 3.57405, 3.58435, 3.59465, 3.60495, 3.61524, 3.62554, 3.63584, 3.64614, 3.65644, 3.66673, 3.67703, 3.68733, 3.69763, 3.71041, 3.72113, 3.72997, 3.73882, 3.74912, 3.75936, 3.76951, 3.7791, 3.78865, 3.79787, 3.80709, 3.8161, 3.82509, 3.83409, 3.84308, 3.85207, 3.86107, 3.87006, 3.87901, 3.88831, 3.89824, 3.90887, 3.91951, 3.93012, 3.94073, 3.95138, 3.96184, 3.97226, 3.98268, 3.99311, 4.0032, 4.01221, 4.01944, 4.02668, 4.03286, 4.03874, 4.04383, 4.0488, 4.05377, 4.05873, 4.06312, 4.06753, 4.07333, 4.08117, 4.08904, 4.09911, 4.11111, 4.13802, 4.16831] V  V_rangeCell=[2.25, Inf] V  R0_vecCell=[.02095, .01921, .01774, .0166, .01557, .01469, .01398, .01338, .01283, .01239, .01196, .01155, .01116, .01079, .01042, .01007, .00974, .00949, .00924, .009, .00876, .00855, .00843, .00832, .00826, .00825, .00825, .00826, .00827, .00828, .0083, .00834, .00838, .00842, .00848, .00855, .00863, .00871, .00879, .00887, .00895, .00903, .00911, .00918, .00925, .00931, .00938, .00946, .00953, .00961, .00968, .00976, .00991, .01, .01003, .01006, .01013, .01022, .0103, .01037, .01043, .01049, .01055, .01061, .01066, .01072, .01077, .01082, .01088, .01093, .01099, .01105, .01114, .01125, .01136, .01148, .01161, .01175, .01188, .01202, .01215, .01228, .01241, .01253, .01261, .01269, .01275, .0128, .01285, .01289, .01294, .01298, .01296, .01292, .01292, .01288, .01282, .0128, .01232, .01214, .00952] Ohm  AHCell=4.493 A*hr  extrapolation_optionCell=simscape.enum.extrapolation.nearest  P=1  S=13  iCell_specify=off  iCell_priority=None  iCell=0 A  iCell_nominal_specify=off  iCell_nominal_value=1  iCell_nominal_unit=A  vCell_specify=off  vCell_priority=None  vCell=0 V  vCell_nominal_specify=off  vCell_nominal_value=1  vCell_nominal_unit=V  socCell_specify=on  socCell_priority=High  socCell=0.08  socCell_nominal_specify=off  socCell_nominal_value=1  socCell_nominal_unit=1  numCyclesCell_specify=off  numCyclesCell_priority=High  numCyclesCell=0  numCyclesCell_nominal_specify=off  numCyclesCell_nominal_value=1  numCyclesCell_nominal_unit=1  vParallelAssembly_specify=off  vParallelAssembly_priority=None  vParallelAssembly=repmat(0, 13, 1) V  vParallelAssembly_nominal_specify=off  vParallelAssembly_nominal_value=1  vParallelAssembly_nominal_unit=V  socParallelAssembly_specify=off  socParallelAssembly_priority=None  socParallelAssembly=repmat(1, 13, 1)  socParallelAssembly_nominal_specify=off  socParallelAssembly_nominal_value=1  socParallelAssembly_nominal_unit=1
      settings: InternalSimscapePortConfiguration="{\"Bottom\":[{\"id\":\"n\",\"label\":\"-\",\"type\":\"foundation.electrical.electrical\"}],\"Left\":[],\"Right\":[],\"Top\":[{\"id\":\"p\",\"label\":\"+\",\"type\":\"foundation.electrical.electrical\"}]}"
  Module2_outputs : SimscapeProbe  BoundBlock=140  Variables="{\"iCell\":{\"Probing\":\"ON\"},\"numCyclesCell\":{\"Probing\":\"ON\"},\"socCell\":{\"Probing\":\"ON\"},\"socParallelAssembly\":{\"Probing\":\"ON\"},\"vCell\":{\"Probing\":\"ON\"},\"vParallelAssembly\":{\"Probing\":\"ON\"}}"
  Module3_outputs : SimscapeProbe  BoundBlock=142  Variables="{\"iCell\":{\"Probing\":\"ON\"},\"numCyclesCell\":{\"Probing\":\"ON\"},\"socCell\":{\"Probing\":\"ON\"},\"socParallelAssembly\":{\"Probing\":\"ON\"},\"vCell\":{\"Probing\":\"ON\"},\"vParallelAssembly\":{\"Probing\":\"ON\"}}"
  Module4_outputs : SimscapeProbe  BoundBlock=144  Variables="{\"iCell\":{\"Probing\":\"ON\"},\"numCyclesCell\":{\"Probing\":\"ON\"},\"socCell\":{\"Probing\":\"ON\"},\"socParallelAssembly\":{\"Probing\":\"ON\"},\"vCell\":{\"Probing\":\"ON\"},\"vParallelAssembly\":{\"Probing\":\"ON\"}}"
  Module5_outputs : SimscapeProbe  BoundBlock=146  Variables="{\"iCell\":{\"Probing\":\"ON\"},\"numCyclesCell\":{\"Probing\":\"ON\"},\"socCell\":{\"Probing\":\"ON\"},\"socParallelAssembly\":{\"Probing\":\"ON\"},\"vCell\":{\"Probing\":\"ON\"},\"vParallelAssembly\":{\"Probing\":\"ON\"}}"
  NewModule : Batteries_lib/Modules/ModuleType1  SOC_vecCell=[0, .01, .02, .03, .04, .05, .06, .07, .08, .09, .1, .11, .12, .13, .14, .15, .16, .17, .18, .19, .2, .21, .22, .23, .24, .25, .26, .27, .28, .29, .3, .31, .32, .33, .34, .35, .36, .37, .38, .39, .4, .41, .42, .43, .44, .45, .46, .47, .48, .49, .5, .51, .52, .53, .54, .55, .56, .57, .58, .59, .6, .61, .62, .63, .64, .65, .66, .67, .68, .69, .7, .71, .72, .73, .74, .75, .76, .77, .78, .79, .8, .81, .82, .83, .84, .85, .86, .87, .88, .89, .9, .91, .92, .93, .94, .95, .96, .97, .98, .99, 1]  V0_vecCell=[3.17242, 3.18272, 3.19302, 3.20331, 3.21361, 3.22391, 3.23421, 3.24451, 3.25481, 3.2651, 3.2754, 3.2857, 3.296, 3.3063, 3.31659, 3.32689, 3.33719, 3.34749, 3.35779, 3.36809, 3.37838, 3.38868, 3.39898, 3.40928, 3.41958, 3.42988, 3.44017, 3.45047, 3.46077, 3.47107, 3.48137, 3.49166, 3.50196, 3.51226, 3.52256, 3.53286, 3.54316, 3.55345, 3.56375, 3.57405, 3.58435, 3.59465, 3.60495, 3.61524, 3.62554, 3.63584, 3.64614, 3.65644, 3.66673, 3.67703, 3.68733, 3.69763, 3.71041, 3.72113, 3.72997, 3.73882, 3.74912, 3.75936, 3.76951, 3.7791, 3.78865, 3.79787, 3.80709, 3.8161, 3.82509, 3.83409, 3.84308, 3.85207, 3.86107, 3.87006, 3.87901, 3.88831, 3.89824, 3.90887, 3.91951, 3.93012, 3.94073, 3.95138, 3.96184, 3.97226, 3.98268, 3.99311, 4.0032, 4.01221, 4.01944, 4.02668, 4.03286, 4.03874, 4.04383, 4.0488, 4.05377, 4.05873, 4.06312, 4.06753, 4.07333, 4.08117, 4.08904, 4.09911, 4.11111, 4.13802, 4.16831] V  V_rangeCell=[2.25, Inf] V  R0_vecCell=[.02095, .01921, .01774, .0166, .01557, .01469, .01398, .01338, .01283, .01239, .01196, .01155, .01116, .01079, .01042, .01007, .00974, .00949, .00924, .009, .00876, .00855, .00843, .00832, .00826, .00825, .00825, .00826, .00827, .00828, .0083, .00834, .00838, .00842, .00848, .00855, .00863, .00871, .00879, .00887, .00895, .00903, .00911, .00918, .00925, .00931, .00938, .00946, .00953, .00961, .00968, .00976, .00991, .01, .01003, .01006, .01013, .01022, .0103, .01037, .01043, .01049, .01055, .01061, .01066, .01072, .01077, .01082, .01088, .01093, .01099, .01105, .01114, .01125, .01136, .01148, .01161, .01175, .01188, .01202, .01215, .01228, .01241, .01253, .01261, .01269, .01275, .0128, .01285, .01289, .01294, .01298, .01296, .01292, .01292, .01288, .01282, .0128, .01232, .01214, .00952] Ohm  AHCell=4.493 A*hr  extrapolation_optionCell=simscape.enum.extrapolation.nearest  P=1  S=13  iCell_specify=off  iCell_priority=None  iCell=0 A  iCell_nominal_specify=off  iCell_nominal_value=1  iCell_nominal_unit=A  vCell_specify=off  vCell_priority=None  vCell=0 V  vCell_nominal_specify=off  vCell_nominal_value=1  vCell_nominal_unit=V  socCell_specify=on  socCell_priority=High  socCell=0.08  socCell_nominal_specify=off  socCell_nominal_value=1  socCell_nominal_unit=1  numCyclesCell_specify=off  numCyclesCell_priority=High  numCyclesCell=0  numCyclesCell_nominal_specify=off  numCyclesCell_nominal_value=1  numCyclesCell_nominal_unit=1  vParallelAssembly_specify=off  vParallelAssembly_priority=None  vParallelAssembly=repmat(0, 13, 1) V  vParallelAssembly_nominal_specify=off  vParallelAssembly_nominal_value=1  vParallelAssembly_nominal_unit=V  socParallelAssembly_specify=off  socParallelAssembly_priority=None  socParallelAssembly=repmat(1, 13, 1)  socParallelAssembly_nominal_specify=off  socParallelAssembly_nominal_value=1  socParallelAssembly_nominal_unit=1
      settings: InternalSimscapePortConfiguration="{\"Bottom\":[{\"id\":\"n\",\"label\":\"-\",\"type\":\"foundation.electrical.electrical\"}],\"Left\":[],\"Right\":[],\"Top\":[{\"id\":\"p\",\"label\":\"+\",\"type\":\"foundation.electrical.electrical\"}]}"
  NewModule_outputs : SimscapeProbe  BoundBlock=148  Variables="{\"iCell\":{\"Probing\":\"ON\"},\"numCyclesCell\":{\"Probing\":\"ON\"},\"socCell\":{\"Probing\":\"ON\"},\"socParallelAssembly\":{\"Probing\":\"ON\"},\"vCell\":{\"Probing\":\"ON\"},\"vParallelAssembly\":{\"Probing\":\"ON\"}}"
  iCellMux : Mux  Inputs=5
  numCyclesCellMux : Mux  Inputs=5
  socCellMux : Mux  Inputs=5
  socParallelAssemblyMux : Mux  Inputs=5
  vCellMux : Mux  Inputs=5
  vParallelAssemblyMux : Mux  Inputs=5
  + : PMIOPort  Side=Left
  - : PMIOPort  Port=2  Side=Right
  iCell : Outport
  numCyclesCell : Outport  Port=2
  socCell : Outport  Port=3
  socParallelAssembly : Outport  Port=4
  vCell : Outport  Port=5
  vParallelAssembly : Outport  Port=6
  wires:
  NewModule_outputs/1 -> [iCell1]
  iCellMux/1 -> iCell/1
  [iCell1] -> iCellMux/1
  NewModule_outputs/2 -> [numCyclesCell1]
  numCyclesCellMux/1 -> numCyclesCell/1
  [numCyclesCell1] -> numCyclesCellMux/1
  NewModule_outputs/3 -> [socCell1]
  socCellMux/1 -> socCell/1
  [socCell1] -> socCellMux/1
  NewModule_outputs/4 -> [socParallelAssembly1]
  socParallelAssemblyMux/1 -> socParallelAssembly/1
  [socParallelAssembly1] -> socParallelAssemblyMux/1
  NewModule_outputs/5 -> [vCell1]
  vCellMux/1 -> vCell/1
  [vCell1] -> vCellMux/1
  NewModule_outputs/6 -> [vParallelAssembly1]
  vParallelAssemblyMux/1 -> vParallelAssembly/1
  [vParallelAssembly1] -> vParallelAssemblyMux/1
  Module2_outputs/1 -> [iCell2]
  [iCell2] -> iCellMux/2
  Module2_outputs/2 -> [numCyclesCell2]
  [numCyclesCell2] -> numCyclesCellMux/2
  Module2_outputs/3 -> [socCell2]
  [socCell2] -> socCellMux/2
  Module2_outputs/4 -> [socParallelAssembly2]
  [socParallelAssembly2] -> socParallelAssemblyMux/2
  Module2_outputs/5 -> [vCell2]
  [vCell2] -> vCellMux/2
  Module2_outputs/6 -> [vParallelAssembly2]
  [vParallelAssembly2] -> vParallelAssemblyMux/2
  Module3_outputs/1 -> [iCell3]
  [iCell3] -> iCellMux/3
  Module3_outputs/2 -> [numCyclesCell3]
  [numCyclesCell3] -> numCyclesCellMux/3
  Module3_outputs/3 -> [socCell3]
  [socCell3] -> socCellMux/3
  Module3_outputs/4 -> [socParallelAssembly3]
  [socParallelAssembly3] -> socParallelAssemblyMux/3
  Module3_outputs/5 -> [vCell3]
  [vCell3] -> vCellMux/3
  Module3_outputs/6 -> [vParallelAssembly3]
  [vParallelAssembly3] -> vParallelAssemblyMux/3
  Module4_outputs/1 -> [iCell4]
  [iCell4] -> iCellMux/4
  Module4_outputs/2 -> [numCyclesCell4]
  [numCyclesCell4] -> numCyclesCellMux/4
  Module4_outputs/3 -> [socCell4]
  [socCell4] -> socCellMux/4
  Module4_outputs/4 -> [socParallelAssembly4]
  [socParallelAssembly4] -> socParallelAssemblyMux/4
  Module4_outputs/5 -> [vCell4]
  [vCell4] -> vCellMux/4
  Module4_outputs/6 -> [vParallelAssembly4]
  [vParallelAssembly4] -> vParallelAssemblyMux/4
  Module5_outputs/1 -> [iCell5]
  [iCell5] -> iCellMux/5
  Module5_outputs/2 -> [numCyclesCell5]
  [numCyclesCell5] -> numCyclesCellMux/5
  Module5_outputs/3 -> [socCell5]
  [socCell5] -> socCellMux/5
  Module5_outputs/4 -> [socParallelAssembly5]
  [socParallelAssembly5] -> socParallelAssemblyMux/5
  Module5_outputs/5 -> [vCell5]
  [vCell5] -> vCellMux/5
  Module5_outputs/6 -> [vParallelAssembly5]
  [vParallelAssembly5] -> vParallelAssemblyMux/5
  connections:
  Module2/LConn1 -- NewModule/RConn1
  Module3/LConn1 -- Module2/RConn1
  Module4/LConn1 -- Module3/RConn1
  Module5/LConn1 -- Module4/RConn1
  NewModule/LConn1 -- +/RConn1
  Module5/RConn1 -- -/RConn1
